simulink model "TestCase5_FromAero_RealWindTester"  (R2023a)
settings: Solver=ode4  StartTime=0.0  StopTime=120  FixedStep=0.01  RelTol=1e-3
values from neighbouring files (symbols this model uses):
  a0_All = [a0_s2 a0_s3 a0_s4 a0_s5]    [aeroProperties.m]
  aircraftMass = sum(componentMassesAndGeom(:,1))    [aircraftMassModel.m]
  AR_All = [AR_s2 AR_s3 AR_s4 AR_s5]    [DefineAircraftGeometry.m]
  c_All = [c_s2 c_s3 c_s4 c_s5]    [DefineAircraftGeometry.m]
  CD0_All = [CD0_s2 CD0_s3 CD0_s4 CD0_s5]    [aeroProperties.m]
  CDa_All = [CDa_s2 CDa_s3 CDa_s4 CDa_s5]    [aeroProperties.m]
  CG = [x_B_B_cmR y_B_B_cmR z_B_B_cmR]    [aircraftMassModel.m]
  CL0_All = [CL0_s2 CL0_s3 CL0_s4 CL0_s5]    [aeroProperties.m]
  CL_alpha_All = [CL_alpha_s2 CL_alpha_s3 CL_alpha_s4 CL_alpha_s5]    [aeroProperties.m]
  CM0_All = [CM0_s2 CM0_s3 CM0_s4 CM0_s5]    [aeroProperties.m]
  CMa_All = [CMa_s2 CMa_s3 CMa_s4 CMa_s5]    [aeroProperties.m]
  e_All = [e_s2 e_s3 e_s4 e_s5]    [aeroProperties.m]
  iAll = [i_s2 i_s3 i_s4 i_s5]    [aeroProperties.m]
  n_s2 = [0; 0; -1]    [aeroProperties.m]
  n_s3 = [0; 1; 0]    [aeroProperties.m]
  n_s4 = [0; 0; -1]    [aeroProperties.m]
  n_s5 = [0; 0; -1]    [aeroProperties.m]
  nAll = [n_s2 n_s3 n_s4 n_s5]    [aeroProperties.m]
  S_All = [S_s2 S_s3 S_s4 S_s5]    [DefineAircraftGeometry.m]
  x_horStab_B_B = [horStab_xLoc+0.25*c_s2 horStab_yLoc horStab_zLoc]    [aircraftMassModel.m]
  x_leftWingandServo_B_B = [leftWingandServo_xLoc+0.25*c_s5 leftWingandServo_yLoc leftWingandServo_zLoc]    [aircraftMassModel.m]
  x_rightWingandServo_B_B = [rightWingandServo_xLoc+0.25*c_s4 rightWingandServo_yLoc rightWingandServo_zLoc]    [aircraftMassModel.m]
  x_vertStab_B_B = [vertStab_xLoc+0.25*c_s3 vertStab_yLoc vertStab_zLoc]    [aircraftMassModel.m]
undefined symbols (not defined in the file or in its folder): earthRadius
libraries: matrix_library x6, simulink_extras x4, aerolibfltsims x2, aerolibtransform2 x1, aerolibutil x1, neural x1, sharedtransform x1
settings Model: Creator=fahee  LastModifiedBy=fahee

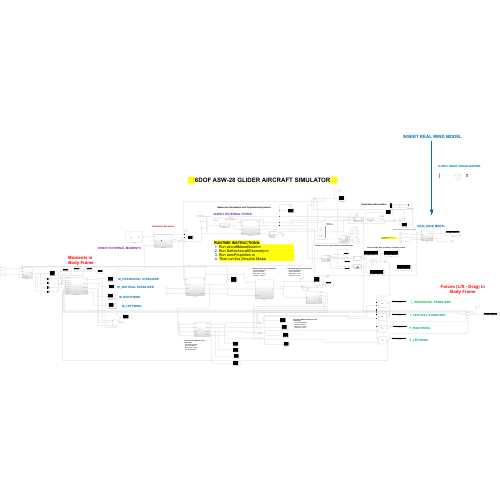
[thumbnail: Simulink's stored preview of the top-level diagram]
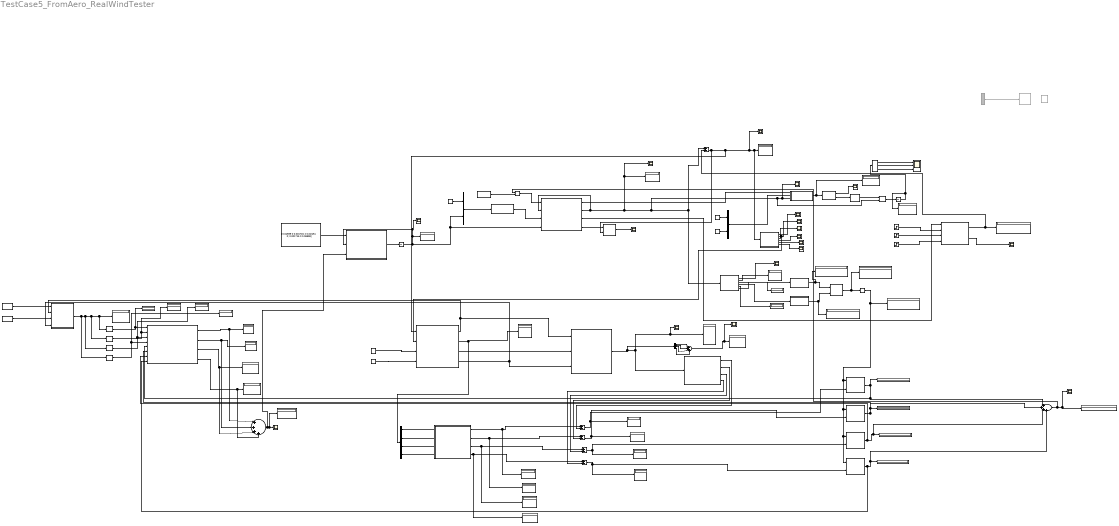
== system TestCase5_FromAero_RealWindTester ==
  note: FLIGHT GEAR VISUALIZATION
  note: v_N = C_N/B*v_B
  note: pure AKA null quaternion
      | vector part comes from rotational dynamics (omega)
  note: intersection of equator and prime meridian
  note: INSERT EXTERNAL FORCE
  note: 6DOF ASW-28 GLIDER AIRCRAFT SIMULATOR
  note: F_HORIZONTAL STABILIZER
  note: w_B/I
  note: w_B/I_dot
  note: Rotational Dynamics
  note: Translational Kinematics
  note: Latitude and Longitude (NED)
  note: Quaternion Kinematics and Translational Dynamics
  note: Calculate Airspeed, Angle of Attack and SideSlip Angle
  note: Calculate FORCE in Wind for each component
      | - Horzontal Stabilizer
      | - Vertical Stabilizer
      | - Right Wing + Servo
      | - Left Wing + Servo
  note: Calculate Drag for each component:
      | - Horzontal Stabilizer
      | - Vertical Stabilizer
      | - Right Wing + Servo
      | - Left Wing + Servo
  note: Calculate DCMs, Body to Stability and Stability to Wind
  note: Forces (Lift - Drag) in Body Frame
  note: F_VERTICAL STABILIZER
  note: F_RIGHTWING
  note: F_LEFTWING
  note: M_HORIZONTAL STABILIZER
  note: Moments in
      | Body Frame
  note: M_LEFTWING
  note: M_RIGHTWING
  note: M_VERTICAL STABILIZER
  note: Calculate Lift in Wind for each component
      | - Horzontal Stabilizer
      | - Vertical Stabilizer
      | - Right Wing + Servo
      | - Left Wing + Servo
  note: INSERT EXTERNAL MOMENTS
  note: w_B/I
  note: Specific Force = F_B/aircraftMass
  note: Calculate Lift for each component:
      | - Horzontal Stabilizer
      | - Vertical Stabilizer
      | - Right Wing + Servo
      | - Left Wing + Servo
  note: Add wind in NED as step input (set to 0 as default)
  note: INSERT REAL WIND MODEL
  note: Enter Wind Velocity, x, y z components
  note: RUNTIME INSTRUCTIONS:
      | Run aircraftMassModel.m
      | Run DefineAircraftGeometry.m
      | Run aeroProperties.m
      | Then run this Simulink Model
  note: REAL WIND MODEL
  AircraftMass_kg : Constant  Value=aircraftMass/1000
  Body2Stability : MATLAB Function  TreatAsAtomicUnit=on
  C_B/W : Display
  C_W/B : Display
  Calc Vinf alpha and beta : Subsystem
  Calc Vinf alpha and beta - with wind : Subsystem
  Calcualte v_BA_NED : Subsystem
  Calculate DRAG : Subsystem
  Calculate LIFT : Subsystem
  Constant : Constant  Value=iAll
  Constant1 : Constant  Value=nAll
  Constant17 : Constant  Value=CM0_All
  Constant18 : Constant  Value=CMa_All
  DRAG : Display
  Demux : Demux  Outputs=3
  Demux1 : Demux
  Demux2 : Demux
  Direction Cosine Matrix ECEF to NED : aerolibtransform2/Direction Cosine Matrix ECEF to NED
  Display{,1..4,7,14} (7 alike) : Display
  Divide4 : Product  Inputs=*/
  ECEF to LLA : Subsystem
  F_HorStab_Body : Display
  F_LeftWing_Body : Display
  F_RightWing_Body : Display
  F_VertStab_Body : Display
  FlightGear Preconfigured 6DoF Animation : aerolibfltsims/FlightGear Preconfigured 6DoF Animation  Commented=on  xFlightGearVersion=v2019.1  DestinationIpAddress=127.0.0.1  DestinationPort=5502  SampleTime=1/30  packetVersion=24
  Force_HorStab_WindFrame : Display
  Force_LeftWing_Wind : Display
  Force_RightWing_Wind : Display
  Force_VertStab_WindFrame : Display
  Generate Run Script : aerolibfltsims/Generate Run Script  Commented=on  Architecture=Win64  dataFlow=Send  GeometryModelName=c172p  AirportId=KSFO  RunwayId=10L  InitialAltitude=7224  InitialHeading=113  OffsetDistance=4.72  OffsetAzimuth=0  InstallScenery=off  DisableShaders=on  OriginAddress=127.0.0.1  DestinationPort=5502  OriginPort=5505  LocalAddress=127.0.0.1  OutputFileName=runfg.bat  FlightGearBaseDirectory=C:\Program Files\FlightGear 2020.3
  Inertia Matrix : Constant  Value=[0.04939 0 0.001715; 0 0.02151 0; 0.001715 0 0.06998]
  Integrator : Integrator  InitialCondition=[0 0 0]
  Integrator3 : Integrator  InitialCondition=[earthRadius,0,0]
  LIFT : Display
  L_HorStab_Wind : Display
  L_LeftWing_Wind : Display
  L_RightWing_Wind : Display
  L_VertStab_Wind : Display
  Lift_Wind : Subsystem
  MATLAB Function1 : MATLAB Function  TreatAsAtomicUnit=on
  M_LeftWing_Wind : Display
  M_RightWing_Wind : Display
  M_horstab_wind : Display
  M_vertstab_wind : Display
  Matrix Multiply3 : Product  Multiplication=Matrix(*)
  Moment_HorStab_BodyFrame : Display
  Moment_LeftWing_BodyFrame : Display
  Moment_RightWing_BodyFrame : Display
  Moment_VertStab_BodyFrame : Display
  Moment_Wind : Subsystem
  Moment_WindFrame : Display
  Moments Wind to Body : Subsystem
  Mux2 : Mux  Commented=on  Inputs=2
  Mux3 : Mux  Inputs=2
  Mux6 : Mux  Inputs=2
  Product{1,10..13} (5 alike) : Product  Multiplication=Matrix(*)
  Real Wind : Subsystem
  Rotational Dynamics : Subsystem
  Rotational Kinematics : Subsystem
  Scope{,1,4..11,13..14} (12 alike) : Scope
  Scope_x_B/E_E_latlonmethod : Scope  NumInputPorts=3
  Selector : Selector  InputPortWidth=4  IndexOptions=Index vector (dialog)  Indices=[1]  OutputSizes=1
  Selector1 : Selector  InputPortWidth=4  IndexOptions=Index vector (dialog)  Indices=[2]  OutputSizes=1
  Selector2 : Selector  InputPortWidth=4  IndexOptions=Index vector (dialog)  Indices=[3]  OutputSizes=1
  Selector3 : Selector  InputPortWidth=4  IndexOptions=Index vector (dialog)  Indices=[4]  OutputSizes=1
  Split to Drag For Each Control Surface : Subsystem
  Subtract{,1..4} (5 alike) : Sum  Inputs=+-
  Sum : Sum  Inputs=|++++
  Sum2 : Sum  Inputs=|++++
  Sum3 : Sum  Inputs=|++++
  Translational Dynamics : Subsystem
  Transpose3 : Math  Operator=transpose
  V_Wind_X : Step  Time=0  After=0  SampleTime=0
  V_Wind_Y : Step  Time=0  After=0  SampleTime=0
  V_Wind_Z : Step  Time=0  After=0  SampleTime=0
  VectTransform - Body to ECEF : Subsystem
  Vinf : Display
  Vinf alpha beta : Scope
  Wind in Body Frame : Display
  angle of attack : Display
  lat-lon-altitude : Scope
  latitude : Constant  Value=0
  longitude : Constant  Value=0
  qw1 : Constant  Value=0
  sideslip : Display
  v_B/E_B - no Wind : Display
  v_BA_B : Scope
  v_BA_B - subtracting Wind : Display
  v_Body : Scope
  v_NED : Scope
  x_B/E_E : Display
  x_B/Edot : Scope
  wires:
  Direction Cosine Matrix ECEF to NED/1 -> Matrix Multiply3/1
  Translational Dynamics/1(eul_N/B_out) -> VectTransform - Body to ECEF/1(eulAngle_N/B)
  latitude/1 -> Mux6/1
  Mux6/1 -> VectTransform - Body to ECEF/2(lat-lon)
  Matrix Multiply3/1 -> Integrator3/1
  Integrator/1 -> Translational Dynamics/4(w_B/E), Mux3/2, Display/1, Scope/1, Rotational Dynamics/2(w_B/I)
  qw1/1 -> Mux3/1
  VectTransform - Body to ECEF/1(rECEF) -> ECEF to LLA/1(rECEF), x_B/E_E/1
  longitude/1 -> Mux6/2
  Integrator3/1 -> Demux/1, Display14/1
  Demux/1 -> Scope_x_B/E_E_latlonmethod/1  "x_B/E_E"
  Demux/2 -> Scope_x_B/E_E_latlonmethod/2  "y_B/E_E"
  Demux/3 -> Scope_x_B/E_E_latlonmethod/3  "z_B/E_E"
  Subtract1/1 -> Product10/2, Force_HorStab_WindFrame/1
  Subtract2/1 -> Product11/2, Force_VertStab_WindFrame/1
  Subtract3/1 -> Force_RightWing_Wind/1, Product12/2
  Subtract4/1 -> Product13/2, Force_LeftWing_Wind/1
  Transpose3/1 -> Product13/1, Product12/1, Product11/1, Product10/1, C_B/W/1
  Product10/1 -> Moments Wind to Body/5(F_HorStab_Body), Sum/1, F_HorStab_Body/1
  Product11/1 -> Moments Wind to Body/6(F_VertStab_Body), Sum/2, F_VertStab_Body/1
  Product12/1 -> Sum/3, F_RightWing_Body/1, Moments Wind to Body/7(F_RightWing_Body)
  Product13/1 -> Moments Wind to Body/8(F_LeftWing_Body), Sum/4, F_LeftWing_Body/1
  Selector/1 -> M_horstab_wind/1, Moments Wind to Body/1(M_horstab_wind)
  Selector1/1 -> M_vertstab_wind/1, Moments Wind to Body/2(M_vertstab_wind)
  Selector2/1 -> M_RightWing_Wind/1, Moments Wind to Body/3(M_RightWing_Wind)
  Selector3/1 -> Moments Wind to Body/4(M_LeftWing_Wind), M_LeftWing_Wind/1
  Inertia Matrix/1 -> Rotational Dynamics/1(J)
  Rotational Dynamics/1(w_B/I_dot) -> Integrator/1
  Sum/1 -> Divide4/1, Scope7/1, Display7/1
  Mux3/1 -> Rotational Kinematics/1(qNull)
  ECEF to LLA/1(LLA) -> lat-lon-altitude/1
  ECEF to LLA/2(LatLon) -> Direction Cosine Matrix ECEF to NED/1
  Calculate LIFT/1(alpha) -> Moment_Wind/2(alpha), Calculate DRAG/1(alpha)
  Calculate LIFT/4(LDM_CommonTerm) -> Moment_Wind/4(LDM_CommonTerm), Calculate DRAG/3(LDM_CommonTerm)
  Calculate LIFT/2(Lift) -> LIFT/1, Demux2/1
  Constant1/1 -> Calculate LIFT/3(normalVector)
  Constant/1 -> Calculate LIFT/4(incidenceAngle)
  Calculate DRAG/1(Drag) -> Demux1/1, Split to Drag For Each Control Surface/1(Drag_All), Scope13/1, DRAG/1
  Calculate LIFT/3(CL) -> Calculate DRAG/2(CL)
  Split to Drag For Each Control Surface/1(D_HorStab) -> Subtract1/2
  Split to Drag For Each Control Surface/2(D_VertStab) -> Subtract2/2
  Split to Drag For Each Control Surface/3(D_RightWing) -> Subtract3/2
  Split to Drag For Each Control Surface/4(D_LeftWing) -> Subtract4/2
  Demux2/1 -> Lift_Wind/1(L_HorStab)
  Demux2/2 -> Lift_Wind/2(L_VertStab)
  Demux2/3 -> Lift_Wind/3(L_RightWing)
  Demux2/4 -> Lift_Wind/4(L_LeftWing)
  Lift_Wind/1(L_HorStab_Wind) -> L_HorStab_Wind/1, Subtract1/1
  Lift_Wind/2(L_VertStab_Wind) -> L_VertStab_Wind/1, Subtract2/1
  Lift_Wind/3(L_RightWing_Wind) -> Subtract3/1, L_RightWing_Wind/1
  Lift_Wind/4(L_LeftWing_Wind) -> L_LeftWing_Wind/1, Subtract4/1
  Moment_Wind/1(M_Wind) -> Moment_WindFrame/1, Selector/1, Selector1/1, Selector2/1, Selector3/1
  Constant17/1 -> Moment_Wind/1(CM0)
  Constant18/1 -> Moment_Wind/3(CMa)
  Moments Wind to Body/2(M_vertstab_body) -> Sum3/2, Moment_VertStab_BodyFrame/1
  Moments Wind to Body/3(M_RightWing_body) -> Sum3/3, Moment_RightWing_BodyFrame/1
  Moments Wind to Body/4(M_LeftWing_body) -> Sum3/4, Moment_LeftWing_BodyFrame/1
  Moments Wind to Body/1(M_horstab_body) -> Sum3/1, Moment_HorStab_BodyFrame/1
  Sum3/1 -> Rotational Dynamics/3(M_ext), Display4/1, Scope1/1
  Body2Stability/1(C_SB) -> Display2/1, Product1/2
  Product1/1 -> Transpose3/1, C_W/B/1
  Calc Vinf alpha and beta/2(Vinf) -> Vinf/1
  Calc Vinf alpha and beta/3(beta_deg) -> sideslip/1
  Calc Vinf alpha and beta/1(Vinf_alpha_beta) -> Vinf alpha beta/1
  Calc Vinf alpha and beta/4(alpha_rad) -> Body2Stability/1(alpha)
  Calc Vinf alpha and beta/5(alpha_deg) -> angle of attack/1
  Calc Vinf alpha and beta/6(beta_rad) -> MATLAB Function1/1(beta)
  Mux2/1 -> FlightGear Preconfigured 6DoF Animation/1
  Demux1/1 -> Sum2/1
  Demux1/2 -> Sum2/2
  Demux1/3 -> Sum2/3
  Demux1/4 -> Sum2/4
  Sum2/1 -> Scope14/1, Display1/1
  MATLAB Function1/1(C_WS) -> Display3/1, Product1/1
  AircraftMass_kg/1 -> Divide4/2
  Divide4/1 -> Translational Dynamics/1(F_ext)
  Subtract/1 -> Calcualte v_BA_NED/2(v_BA_B), Calculate LIFT/1(v_BA_B), v_BA_B/1, Calc Vinf alpha and beta - with wind/1(v_B/E), v_BA_B - subtracting Wind/1
  Calc Vinf alpha and beta - with wind/1(Vinf_alpha_beta) -> Scope4/1
  Calc Vinf alpha and beta - with wind/2(Vinf) -> Calculate LIFT/2(mag_v_BA_B), Scope5/1
  Calc Vinf alpha and beta - with wind/3(beta_deg) -> Scope6/1
  Calc Vinf alpha and beta - with wind/4(alpha_rad) -> Scope8/1
  Calc Vinf alpha and beta - with wind/5(alpha_deg) -> Scope9/1
  Calc Vinf alpha and beta - with wind/6(beta_rad) -> Scope10/1
  Real Wind/1(V_Wind_Body_Display) -> Subtract/2, Wind in Body Frame/1
  V_Wind_X/1 -> Real Wind/2(V_Wind_X)
  V_Wind_Y/1 -> Real Wind/3(V_Wind_Y)
  V_Wind_Z/1 -> Real Wind/4(V_Wind_Z)
  Real Wind/2(V_Wind_Body_Plot) -> Scope11/1
  Translational Dynamics/2(v_B/E) -> Translational Dynamics/2(v_B/E_In), v_B/E_B - no Wind/1, v_Body/1, Matrix Multiply3/2, x_B/Edot/1, VectTransform - Body to ECEF/3(x_B/Edot_B), Calc Vinf alpha and beta/1(v_B/E), Subtract/1
  Rotational Kinematics/1(q_B/N) -> Translational Dynamics/3(q_B/N)
  Translational Dynamics/3(C_B/N) -> Real Wind/1(C_B/N)
  Calcualte v_BA_NED/1(v_BA_N) -> v_NED/1
  Translational Dynamics/4(C_N/B) -> Calcualte v_BA_NED/1(C_N/B)

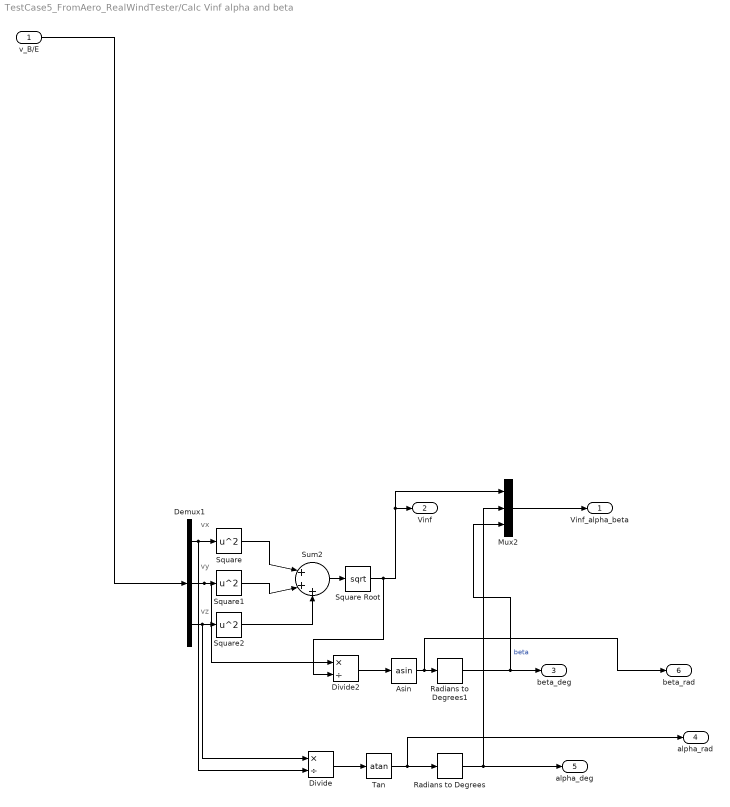
== system TestCase5_FromAero_RealWindTester/Calc Vinf alpha and beta ==
  note: vx
  note: vy
  note: vz
  v_B/E : Inport
  Asin : Trigonometry  Operator=asin
  Demux1 : Demux  Outputs=3
  Divide : Product  Inputs=*/
  Divide2 : Product  Inputs=*/
  Mux2 : Mux  Inputs=3
  Radians to Degrees : simulink_extras/Transformations/Radians to Degrees
  Radians to Degrees1 : simulink_extras/Transformations/Radians to Degrees
  Square : Math  Operator=square
  Square Root : Sqrt
  Square1 : Math  Operator=square
  Square2 : Math  Operator=square
  Sum2 : Sum  Inputs=|+++
  Tan : Trigonometry  Operator=atan
  Vinf_alpha_beta : Outport
  Vinf : Outport  Port=2
  beta_deg : Outport  Port=3
  alpha_rad : Outport  Port=4
  alpha_deg : Outport  Port=5
  beta_rad : Outport  Port=6
  wires:
  Demux1/3 -> Divide/1, Square2/1
  Square/1 -> Sum2/1
  Tan/1 -> alpha_rad/1, Radians to Degrees/1
  Mux2/1 -> Vinf_alpha_beta/1
  Demux1/2 -> Divide2/1, Square1/1
  Radians to Degrees1/1 -> beta_deg/1, Mux2/3  "beta"
  Square1/1 -> Sum2/2
  Divide2/1 -> Asin/1
  Sum2/1 -> Square Root/1
  Asin/1 -> beta_rad/1, Radians to Degrees1/1
  Divide/1 -> Tan/1
  Demux1/1 -> Square/1, Divide/2
  Radians to Degrees/1 -> alpha_deg/1, Mux2/2
  Square2/1 -> Sum2/3
  Square Root/1 -> Divide2/2, Mux2/1, Vinf/1
  v_B/E/1 -> Demux1/1

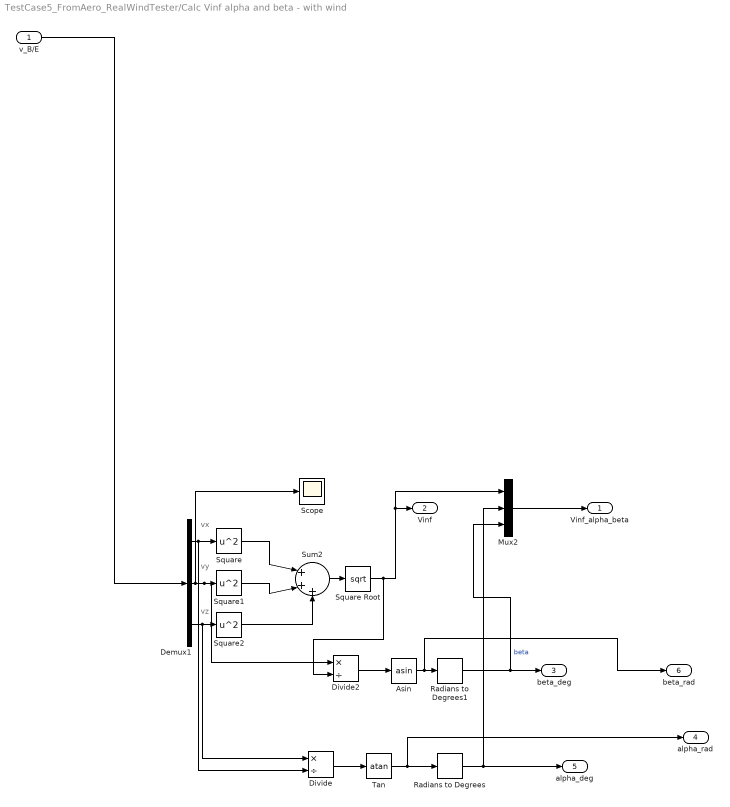
== system TestCase5_FromAero_RealWindTester/Calc Vinf alpha and beta - with wind ==
  note: vx
  note: vy
  note: vz
  v_B/E : Inport
  Asin : Trigonometry  Operator=asin
  Demux1 : Demux  Outputs=3
  Divide : Product  Inputs=*/
  Divide2 : Product  Inputs=*/
  Mux2 : Mux  Inputs=3
  Radians to Degrees : simulink_extras/Transformations/Radians to Degrees
  Radians to Degrees1 : simulink_extras/Transformations/Radians to Degrees
  Scope : Scope
  Square : Math  Operator=square
  Square Root : Sqrt
  Square1 : Math  Operator=square
  Square2 : Math  Operator=square
  Sum2 : Sum  Inputs=|+++
  Tan : Trigonometry  Operator=atan
  Vinf_alpha_beta : Outport
  Vinf : Outport  Port=2
  beta_deg : Outport  Port=3
  alpha_rad : Outport  Port=4
  alpha_deg : Outport  Port=5
  beta_rad : Outport  Port=6
  wires:
  Demux1/3 -> Divide/1, Square2/1
  Square/1 -> Sum2/1
  Tan/1 -> alpha_rad/1, Radians to Degrees/1
  Mux2/1 -> Vinf_alpha_beta/1
  Demux1/2 -> Divide2/1, Square1/1, Scope/1
  Radians to Degrees1/1 -> beta_deg/1, Mux2/3  "beta"
  Square1/1 -> Sum2/2
  Divide2/1 -> Asin/1
  Sum2/1 -> Square Root/1
  Asin/1 -> beta_rad/1, Radians to Degrees1/1
  Divide/1 -> Tan/1
  Demux1/1 -> Square/1, Divide/2
  Radians to Degrees/1 -> alpha_deg/1, Mux2/2
  Square2/1 -> Sum2/3
  Square Root/1 -> Divide2/2, Mux2/1, Vinf/1
  v_B/E/1 -> Demux1/1

== system TestCase5_FromAero_RealWindTester/Calcualte v_BA_NED ==
  C_N/B : Inport
  v_BA_B : Inport  Port=2
  Product24 : Product  Multiplication=Matrix(*)
  v_BA_N : Outport
  wires:
  Product24/1 -> v_BA_N/1
  v_BA_B/1 -> Product24/2
  C_N/B/1 -> Product24/1

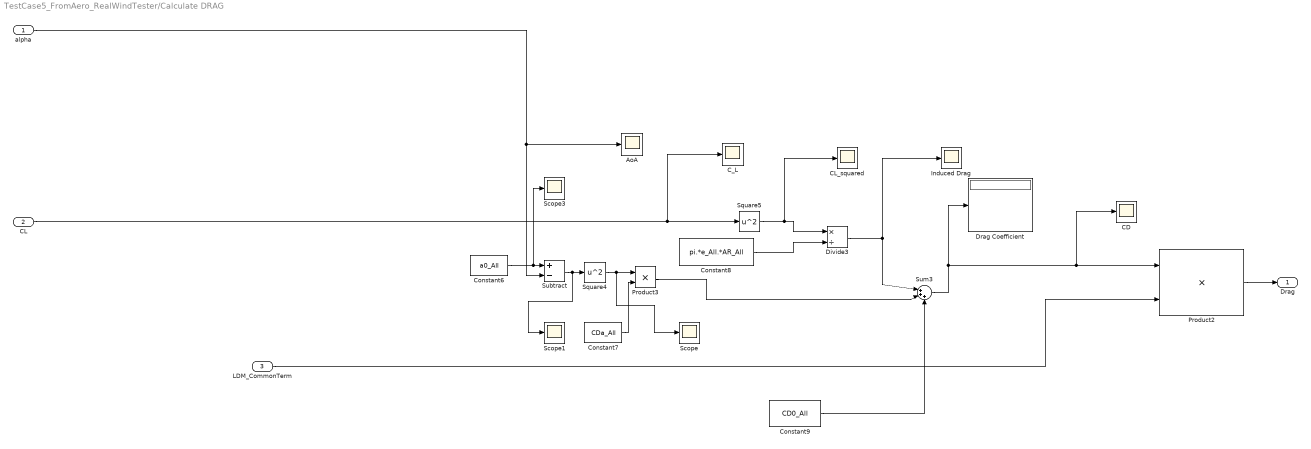
== system TestCase5_FromAero_RealWindTester/Calculate DRAG ==
  alpha : Inport
  CL : Inport  Port=2
  LDM_CommonTerm : Inport  Port=3
  AoA : Scope
  CD : Scope
  CL_squared : Scope
  C_L : Scope
  Constant6 : Constant  Value=a0_All
  Constant7 : Constant  Value=CDa_All
  Constant8 : Constant  Value=pi.*e_All.*AR_All
  Constant9 : Constant  Value=CD0_All
  Divide3 : Product  Inputs=*/
  Drag Coefficient : Display
  Induced Drag : Scope
  Product2 : Product
  Product3 : Product
  Scope : Scope
  Scope1 : Scope
  Scope3 : Scope
  Square4 : Math  Operator=square
  Square5 : Math  Operator=square
  Subtract : Sum  Inputs=+-
  Sum3 : Sum  Inputs=|+++
  Drag : Outport
  wires:
  Subtract/1 -> Scope1/1, Square4/1
  LDM_CommonTerm/1 -> Product2/2
  Constant6/1 -> Scope3/1, Subtract/1
  Constant7/1 -> Product3/2
  Product3/1 -> Sum3/2
  Square4/1 -> Scope/1, Product3/1
  Divide3/1 -> Sum3/1, Induced Drag/1
  Sum3/1 -> Drag Coefficient/1, CD/1, Product2/1
  Constant9/1 -> Sum3/3
  Square5/1 -> CL_squared/1, Divide3/1
  Constant8/1 -> Divide3/2
  Product2/1 -> Drag/1
  alpha/1 -> Subtract/2, AoA/1
  CL/1 -> C_L/1, Square5/1

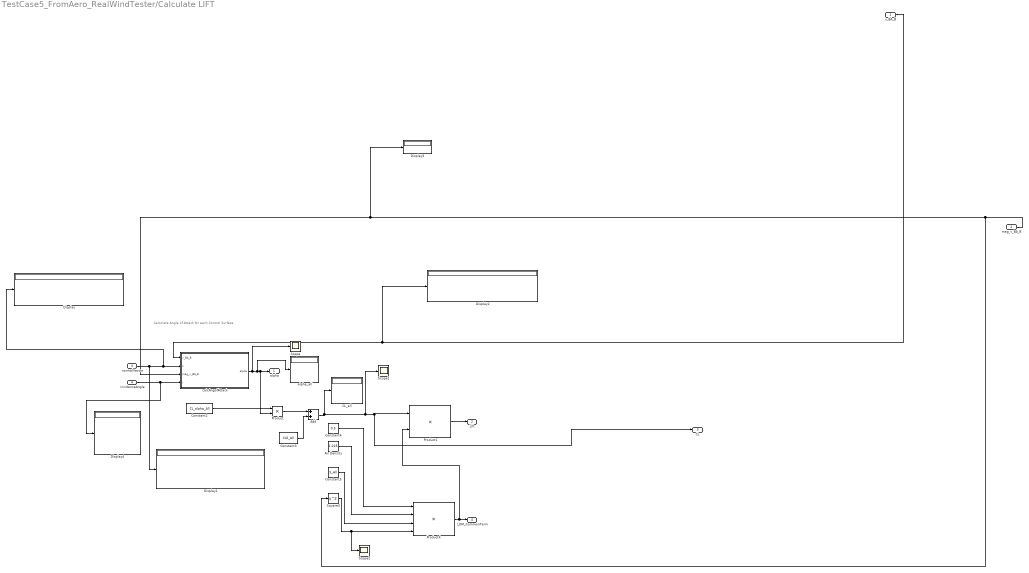
== system TestCase5_FromAero_RealWindTester/Calculate LIFT ==
  note: Calculate Angle of Attack for each Control Surface
  v_BA_B : Inport
  mag_v_BA_B : Inport  Port=2
  normalVector : Inport  Port=3
  incidenceAngle : Inport  Port=4
  Add : Sum
  Air Density : Constant  Value=1.225
  CL_all : Display
  Constant2 : Constant  Value=CL_alpha_All
  Constant3 : Constant  Value=CL0_All
  Constant4 : Constant  Value=0.5
  Constant5 : Constant  Value=S_All
  Display{,1..4} (5 alike) : Display
  Product : Product
  Product1 : Product
  Product4 : Product  Inputs=4
  Scope : Scope
  Scope1 : Scope
  Scope2 : Scope
  Square3 : Math  Operator=square
  alpha_all : Display
  calcAngofAttack : MATLAB Function  TreatAsAtomicUnit=on
  alpha : Outport
  Lift : Outport  Port=2
  CL : Outport  Port=3
  LDM_CommonTerm : Outport  Port=4
  wires:
  Air Density/1 -> Product4/2
  Constant3/1 -> Add/2
  incidenceAngle/1 -> Display4/1, calcAngofAttack/4(i)
  Constant5/1 -> Product4/3
  Constant4/1 -> Product4/1
  Add/1 -> Scope1/1, Product1/1, CL/1, CL_all/1
  normalVector/1 -> Display1/1, Display/1, calcAngofAttack/2(n)
  Square3/1 -> Scope2/1, Product4/4
  Product/1 -> Add/1
  Constant2/1 -> Product/1
  mag_v_BA_B/1 -> Square3/1, Display3/1, calcAngofAttack/3(mag_v_BA_B)
  calcAngofAttack/1(alpha) -> Scope/1, alpha_all/1, alpha/1, Product/2
  Product4/1 -> Product1/2, LDM_CommonTerm/1
  Product1/1 -> Lift/1
  v_BA_B/1 -> Display2/1, calcAngofAttack/1(v_BA_B)

== system TestCase5_FromAero_RealWindTester/ECEF to LLA ==
  note: x_B/Edot_B
  rECEF : Inport
  ECEF Position to LLA : ECEF2LLA  ptype=Custom  R=earthRadius
  Mux4 : Mux  Inputs=2
  altitude : Display
  lat & lon : Display
  LLA : Outport
  LatLon : Outport  Port=2
  wires:
  Mux4/1 -> LLA/1
  ECEF Position to LLA/2 -> Mux4/2, altitude/1
  ECEF Position to LLA/1 -> LatLon/1, Mux4/1, lat & lon/1
  rECEF/1 -> ECEF Position to LLA/1

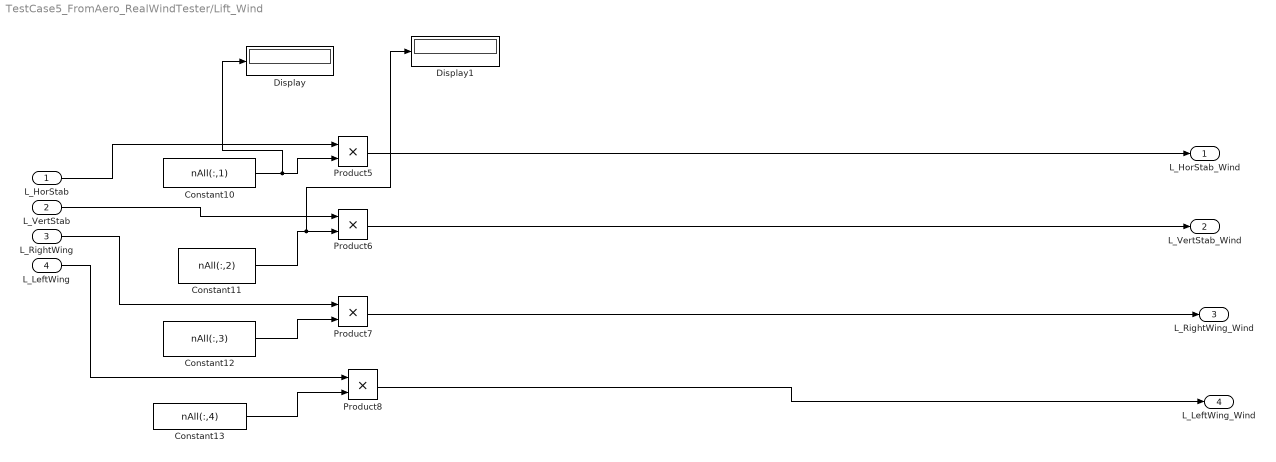
== system TestCase5_FromAero_RealWindTester/Lift_Wind ==
  L_HorStab : Inport
  L_VertStab : Inport  Port=2
  L_RightWing : Inport  Port=3
  L_LeftWing : Inport  Port=4
  Constant10 : Constant  Value=nAll(:,1)
  Constant11 : Constant  Value=nAll(:,2)
  Constant12 : Constant  Value=nAll(:,3)
  Constant13 : Constant  Value=nAll(:,4)
  Display : Display
  Display1 : Display
  Product{5..8} (4 alike) : Product
  L_HorStab_Wind : Outport
  L_VertStab_Wind : Outport  Port=2
  L_RightWing_Wind : Outport  Port=3
  L_LeftWing_Wind : Outport  Port=4
  wires:
  L_LeftWing/1 -> Product8/1
  L_VertStab/1 -> Product6/1
  Constant11/1 -> Display1/1, Product6/2
  Constant10/1 -> Display/1, Product5/2
  Constant13/1 -> Product8/2
  Constant12/1 -> Product7/2
  L_RightWing/1 -> Product7/1
  Product8/1 -> L_LeftWing_Wind/1
  L_HorStab/1 -> Product5/1
  Product7/1 -> L_RightWing_Wind/1
  Product6/1 -> L_VertStab_Wind/1
  Product5/1 -> L_HorStab_Wind/1

== system TestCase5_FromAero_RealWindTester/Moment_Wind ==
  CM0 : Inport
  alpha : Inport  Port=2
  CMa : Inport  Port=3
  LDM_CommonTerm : Inport  Port=4
  Constant19 : Constant  Value=c_All
  Moment Coefficient : Display
  Product14 : Product
  Product15 : Product  Inputs=3
  Sum4 : Sum  Inputs=|++
  M_Wind : Outport
  wires:
  Sum4/1 -> Product15/2, Moment Coefficient/1
  Constant19/1 -> Product15/3
  LDM_CommonTerm/1 -> Product15/1
  alpha/1 -> Product14/2
  CM0/1 -> Sum4/1
  CMa/1 -> Product14/1
  Product15/1 -> M_Wind/1
  Product14/1 -> Sum4/2

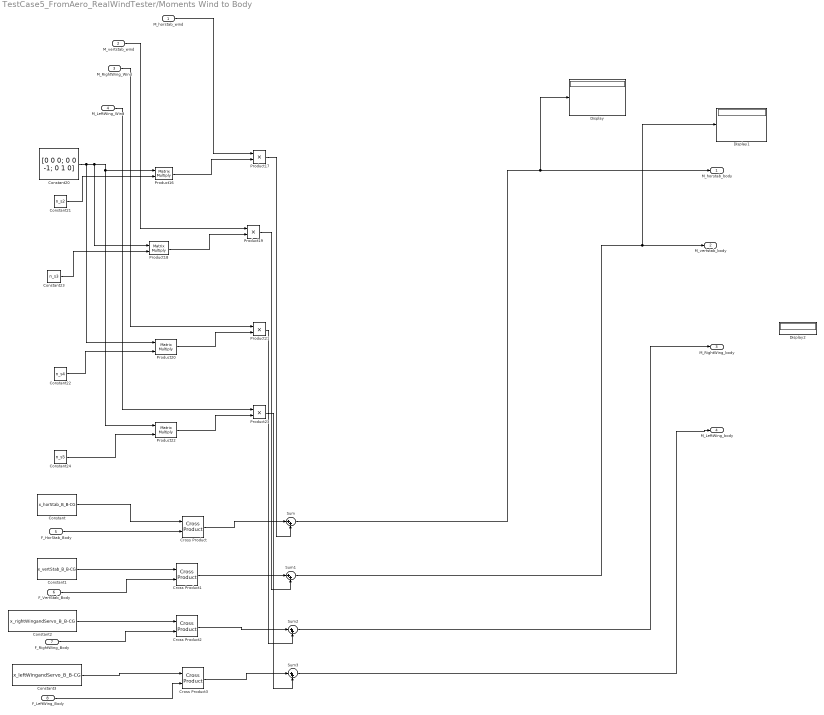
== system TestCase5_FromAero_RealWindTester/Moments Wind to Body ==
  M_horstab_wind : Inport
  M_vertstab_wind : Inport  Port=2
  M_RightWing_Wind : Inport  Port=3
  M_LeftWing_Wind : Inport  Port=4
  F_HorStab_Body : Inport  Port=5
  F_VertStab_Body : Inport  Port=6
  F_RightWing_Body : Inport  Port=7
  F_LeftWing_Body : Inport  Port=8
  Constant : Constant  Value=x_horStab_B_B-CG
  Constant1 : Constant  Value=x_vertStab_B_B-CG
  Constant2 : Constant  Value=x_rightWingandServo_B_B-CG
  Constant20 : Constant  Value=[0 0 0; 0 0 -1; 0 1 0]  VectorParams1D=off  SampleTime=-1
  Constant21 : Constant  Value=n_s2
  Constant22 : Constant  Value=n_s4
  Constant23 : Constant  Value=n_s3
  Constant24 : Constant  Value=n_s5
  Constant3 : Constant  Value=x_leftWingandServo_B_B-CG
  Cross Product{,1..3} (4 alike) : matrix_library/Cross Product
  Display : Display
  Display1 : Display
  Display2 : Display
  Product{16,18,20,22} (4 alike) : Product  Multiplication=Matrix(*)
  Product{17,19,21,23} (4 alike) : Product
  Sum{,1..3} (4 alike) : Sum  Inputs=|++
  M_horstab_body : Outport
  M_vertstab_body : Outport  Port=2
  M_RightWing_body : Outport  Port=3
  M_LeftWing_body : Outport  Port=4
  wires:
  Constant22/1 -> Product20/2
  Constant20/1 -> Product20/1, Product18/1, Product22/1, Product16/1
  Product18/1 -> Product19/2
  Constant21/1 -> Product16/2
  Constant24/1 -> Product22/2
  Constant23/1 -> Product18/2
  M_vertstab_wind/1 -> Product19/1
  Product22/1 -> Product23/2
  Product20/1 -> Product21/2
  M_horstab_wind/1 -> Product17/1
  Product16/1 -> Product17/2
  M_RightWing_Wind/1 -> Product21/1
  M_LeftWing_Wind/1 -> Product23/1
  Constant/1 -> Cross Product/1
  F_HorStab_Body/1 -> Cross Product/2
  Cross Product/1 -> Sum/1
  Product17/1 -> Sum/2
  Sum/1 -> Display/1, M_horstab_body/1
  Constant1/1 -> Cross Product1/1
  F_VertStab_Body/1 -> Cross Product1/2
  Cross Product1/1 -> Sum1/1
  Product19/1 -> Sum1/2
  Sum1/1 -> Display1/1, M_vertstab_body/1
  Constant2/1 -> Cross Product2/1
  F_RightWing_Body/1 -> Cross Product2/2
  Cross Product2/1 -> Sum2/1
  Product21/1 -> Sum2/2
  Sum2/1 -> M_RightWing_body/1
  Constant3/1 -> Cross Product3/1
  F_LeftWing_Body/1 -> Cross Product3/2
  Cross Product3/1 -> Sum3/1
  Product23/1 -> Sum3/2
  Sum3/1 -> M_LeftWing_body/1

== system TestCase5_FromAero_RealWindTester/Real Wind ==
  C_B/N : Inport
  V_Wind_X : Inport  Port=2
  V_Wind_Y : Inport  Port=3
  V_Wind_Z : Inport  Port=4
  Mux4 : Mux  Inputs=3
  Product : Product  Multiplication=Matrix(*)
  V_Wind_Body_Display : Outport
  V_Wind_Body_Plot : Outport  Port=2
  wires:
  Mux4/1 -> V_Wind_Body_Plot/1, Product/2
  Product/1 -> V_Wind_Body_Display/1
  C_B/N/1 -> Product/1
  V_Wind_Y/1 -> Mux4/2
  V_Wind_X/1 -> Mux4/1
  V_Wind_Z/1 -> Mux4/3

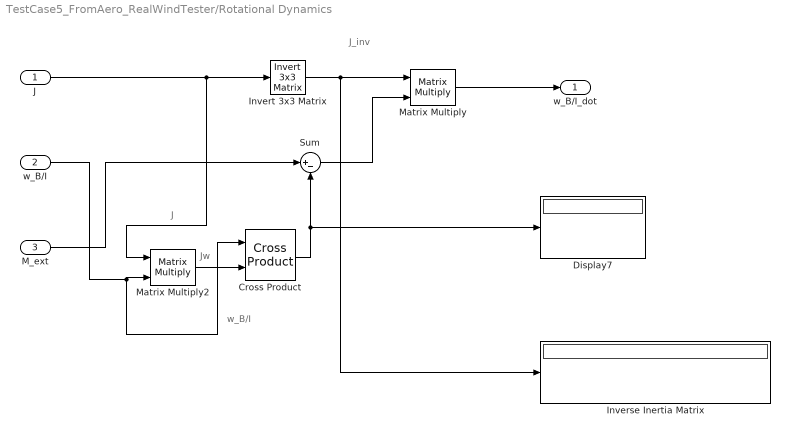
== system TestCase5_FromAero_RealWindTester/Rotational Dynamics ==
  note: J
  note: Jw
  note: J_inv
  note: w_B/I
  J : Inport
  w_B/I : Inport  Port=2
  M_ext : Inport  Port=3
  Cross Product : matrix_library/Cross Product
  Display7 : Display
  Inverse Inertia Matrix : Display
  Invert 3x3 Matrix : aerolibutil/Invert  3x3 Matrix
  Matrix Multiply : Product  Multiplication=Matrix(*)
  Matrix Multiply2 : Product  Multiplication=Matrix(*)
  Sum : Sum  Inputs=|+-
  w_B/I_dot : Outport
  wires:
  Sum/1 -> Matrix Multiply/2
  Cross Product/1 -> Sum/2, Display7/1
  w_B/I/1 -> Cross Product/1, Matrix Multiply2/2
  Matrix Multiply/1 -> w_B/I_dot/1
  J/1 -> Matrix Multiply2/1, Invert 3x3 Matrix/1
  M_ext/1 -> Sum/1
  Matrix Multiply2/1 -> Cross Product/2
  Invert 3x3 Matrix/1 -> Matrix Multiply/1, Inverse Inertia Matrix/1

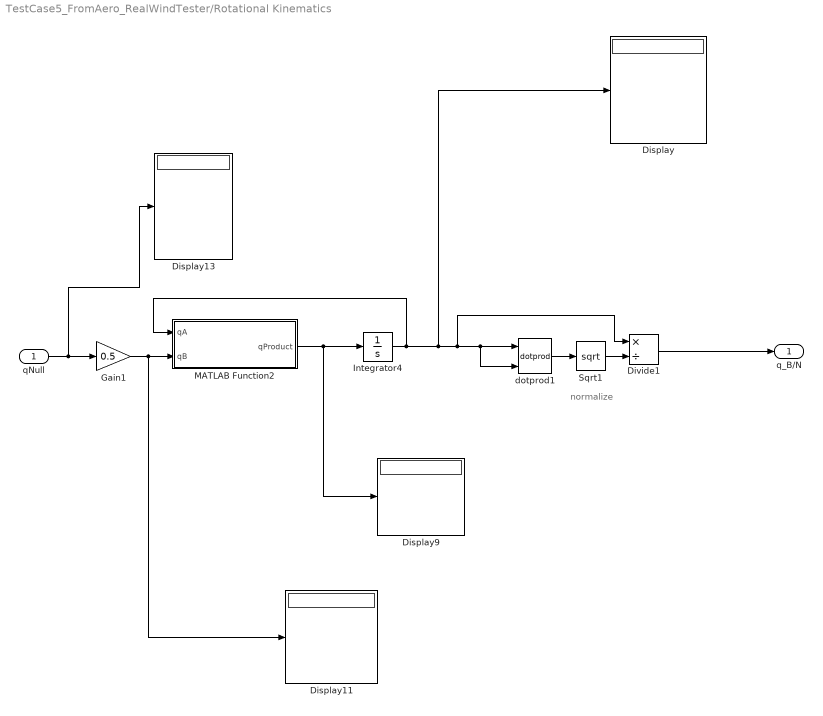
== system TestCase5_FromAero_RealWindTester/Rotational Kinematics ==
  note: normalize
  qNull : Inport
  Display{,9,11,13} (4 alike) : Display
  Divide1 : Product  Inputs=*/
  Gain1 : Gain  Gain=0.5
  Integrator4 : Integrator  InitialCondition=[0.9993 0 -0.03804 0]'
  MATLAB Function2 : MATLAB Function  TreatAsAtomicUnit=on
  Sqrt1 : Sqrt
  dotprod1 : neural/Weight Functions/dotprod
  q_B/N : Outport
  wires:
  Integrator4/1 -> Display/1, Divide1/1, dotprod1/2, dotprod1/1, MATLAB Function2/1(qA)
  dotprod1/1 -> Sqrt1/1
  Gain1/1 -> MATLAB Function2/2(qB), Display11/1
  qNull/1 -> Gain1/1, Display13/1
  MATLAB Function2/1(qProduct) -> Integrator4/1, Display9/1
  Sqrt1/1 -> Divide1/2
  Divide1/1 -> q_B/N/1

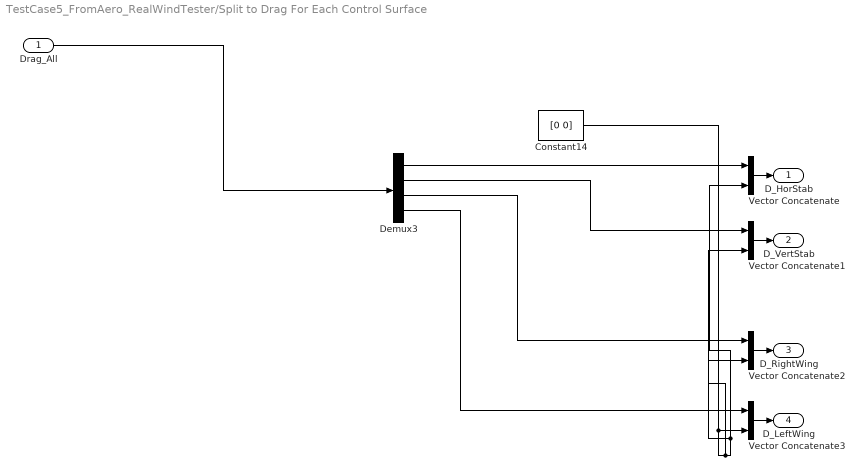
== system TestCase5_FromAero_RealWindTester/Split to Drag For Each Control Surface ==
  Drag_All : Inport
  Constant14 : Constant  Value=[0 0]
  Demux3 : Demux
  Vector Concatenate{,1..3} (4 alike) : Concatenate
  D_HorStab : Outport
  D_VertStab : Outport  Port=2
  D_RightWing : Outport  Port=3
  D_LeftWing : Outport  Port=4
  wires:
  Vector Concatenate1/1 -> D_VertStab/1
  Demux3/3 -> Vector Concatenate2/1
  Constant14/1 -> Vector Concatenate1/2, Vector Concatenate2/2, Vector Concatenate/2, Vector Concatenate3/2
  Vector Concatenate2/1 -> D_RightWing/1
  Demux3/2 -> Vector Concatenate1/1
  Drag_All/1 -> Demux3/1
  Demux3/1 -> Vector Concatenate/1
  Demux3/4 -> Vector Concatenate3/1
  Vector Concatenate/1 -> D_HorStab/1
  Vector Concatenate3/1 -> D_LeftWing/1

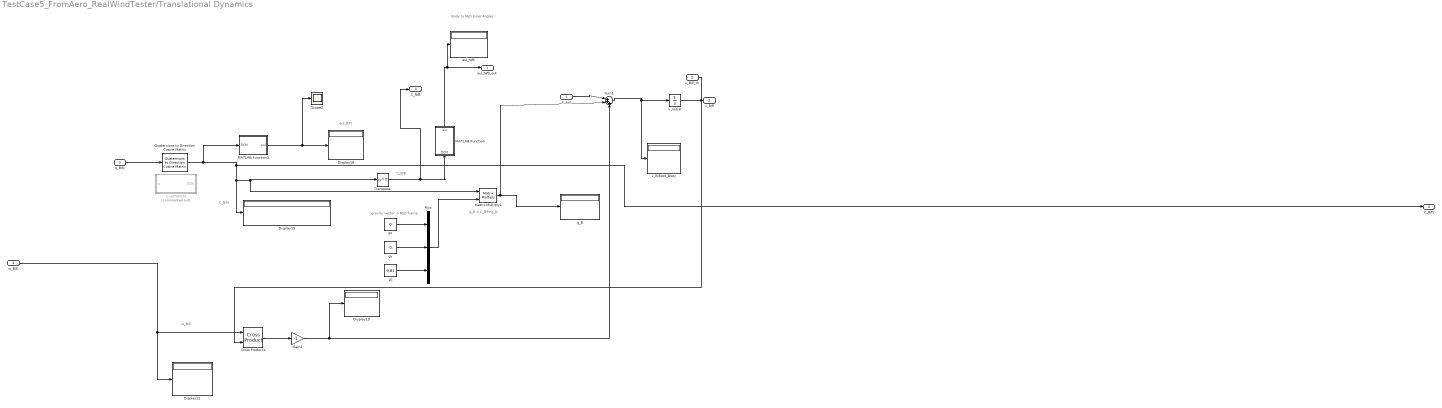
== system TestCase5_FromAero_RealWindTester/Translational Dynamics ==
  note: gravity vector in NED frame
  note: C_N/B
  note: eul_B/N
  note: C_B/N
  note: g_B = C_B/N*g_N
  note: Body to NED Euler Angles
  note: w_B/E
  F_ext : Inport
  v_B/E_In : Inport  Port=2
  q_B/N : Inport  Port=3
  w_B/E : Inport  Port=4
  Cross Product1 : matrix_library/Cross Product
  Display{12,15,18..19} (4 alike) : Display
  Gain2 : Gain  Gain=-1
  MATLAB Function : MATLAB Function  TreatAsAtomicUnit=on
  MATLAB Function3 : MATLAB Function  TreatAsAtomicUnit=on
  Matrix Multiply1 : Product  Multiplication=Matrix(*)
  Mux : Mux  Inputs=3
  QuatToDCM : MATLAB Function  Commented=on  TreatAsAtomicUnit=on
  Quaternions to Direction Cosine Matrix : sharedtransform/Quaternions to  Direction Cosine Matrix  aMode=aMode
      settings: LibrarySourceBlock=|
      | aerolibtransform2/Quaternions to
      | Direction Cosine Matrix
  Scope3 : Scope
  Sum1 : Sum  Inputs=|+++
  Transpose : Math  Operator=transpose
  eul_N/B : Display
  g_B : Display
  gx : Constant  Value=0
  gy : Constant  Value=0
  gz : Constant  Value=9.81
  v_B/Edot_Body : Display
  v_Initial : Integrator  InitialCondition=[13.17 0 -0.1809]
  eul_N/B_out : Outport
  v_B/E : Outport  Port=2
  C_B/N : Outport  Port=3
  C_N/B : Outport  Port=4
  wires:
  Quaternions to Direction Cosine Matrix/1 -> MATLAB Function3/1(DCM), Display15/1, Transpose/1, Matrix Multiply1/1, C_B/N/1
  gy/1 -> Mux/2
  w_B/E/1 -> Cross Product1/1, Display12/1
  Sum1/1 -> v_B/Edot_Body/1, v_Initial/1
  q_B/N/1 -> Quaternions to Direction Cosine Matrix/1
  Gain2/1 -> Sum1/3, Display19/1
  Cross Product1/1 -> Gain2/1
  Transpose/1 -> C_N/B/1, MATLAB Function/1(DCM)
  Mux/1 -> Matrix Multiply1/2
  F_ext/1 -> Sum1/1
  MATLAB Function3/1(eul) -> Display18/1, Scope3/1
  Matrix Multiply1/1 -> Sum1/2, g_B/1
  gx/1 -> Mux/1
  gz/1 -> Mux/3
  v_Initial/1 -> v_B/E/1
  v_B/E_In/1 -> Cross Product1/2
  MATLAB Function/1(eul) -> eul_N/B/1, eul_N/B_out/1

== system TestCase5_FromAero_RealWindTester/VectTransform - Body to ECEF ==
  note: NED to ECEF
  eulAngle_N/B : Inport
  lat-lon : Inport  Port=2
  x_B/Edot_B : Inport  Port=3
  Body to ECEF : Subsystem
  Display : Display
  Integrator1 : Integrator  InitialCondition=[6.371e6 0 1577]
  Scope : Scope
  rECEF : Outport
  wires:
  Integrator1/1 -> Display/1, rECEF/1, Scope/1
  eulAngle_N/B/1 -> Body to ECEF/1(eulAngle_N/B)
  Body to ECEF/1(x_B/Edot_E) -> Integrator1/1
  lat-lon/1 -> Body to ECEF/2(lat-lon)
  x_B/Edot_B/1 -> Body to ECEF/3(x_B/Edot_B)

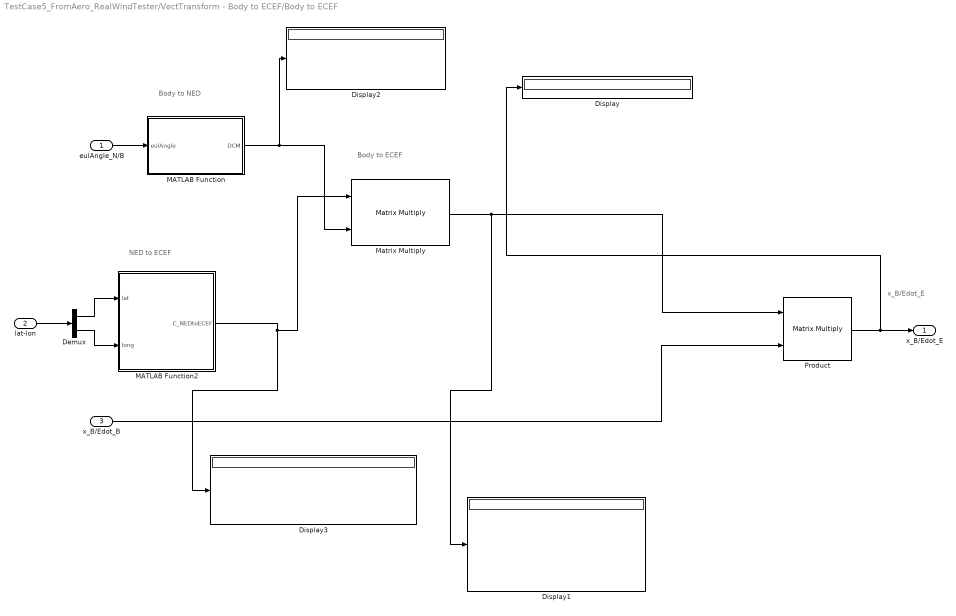
== system TestCase5_FromAero_RealWindTester/VectTransform - Body to ECEF/Body to ECEF ==
  note: NED to ECEF
  note: Body to NED
  note: x_B/Edot_E
  note: Body to ECEF
  eulAngle_N/B : Inport
  lat-lon : Inport  Port=2
  x_B/Edot_B : Inport  Port=3
  Demux : Demux  Outputs=2
  Display{,1..3} (4 alike) : Display
  MATLAB Function : MATLAB Function  TreatAsAtomicUnit=on
  MATLAB Function2 : MATLAB Function  TreatAsAtomicUnit=on
  Matrix Multiply : Product  Multiplication=Matrix(*)
  Product : Product  Multiplication=Matrix(*)
  x_B/Edot_E : Outport
  wires:
  Matrix Multiply/1 -> Display1/1, Product/1
  eulAngle_N/B/1 -> MATLAB Function/1(eulAngle)
  lat-lon/1 -> Demux/1
  x_B/Edot_B/1 -> Product/2
  Product/1 -> Display/1, x_B/Edot_E/1
  MATLAB Function2/1(C_NEDtoECEF) -> Display3/1, Matrix Multiply/1
  MATLAB Function/1(DCM) -> Display2/1, Matrix Multiply/2
  Demux/1 -> MATLAB Function2/1(lat)
  Demux/2 -> MATLAB Function2/2(long)

== matlab function TestCase5_FromAero_RealWindTester/Rotational Kinematics/MATLAB Function2 ==
  data: qA input; qProduct output; qB input
function qProduct = qMult(qA,qB)

%% qMult

% Description: This function is used to perform quaternion multiplication:
%            *************************************************************  
%               qA * qB = qProduct = [ qA(1)*qB(1) - (qA(2:4) dot qB(2:4)); 
%                                     (qA(1)*qB(2:4) + qB(1)*qA(2:4) +
%                                     qA(2:4) cross qB(2:4) ]
%            *************************************************************
% % Aircraft Control and Simulation Third Edition Page 46 Eq 1.8.-4
%
% Inputs:
%  qA - first quaternion in the form [qw qx qy qz]
%  qB - second quaternion in the form [qw qx qy qz]
%
% Output:
%  qProduct - the product of multiplying qA * qB [qw qx qy qz]

% if (norm(qA) ~= 1)
%     error('First quaternion inputted must have length 1. Invalid Quaternion. Try again.')
% end
% 
% if (norm(qB) ~= 1)
%     error('Second quaternion inputted must have length 1. Invalid Quaternion. Try again.')
% end

% Extract scalar components of each of the input quaternions
qA_w = qA(1);
qB_w = qB(1);

% Extract vector components of each of the input quaternions
qA_vect = qA(2:4);
qB_vect = qB(2:4);

% Calculate scalar component of the product of the two quaternions
% Aircraft Control and Simulation Third Edition Page 46 Eq 1.8.-4
qProd_w = (qA_w*qB_w - dot(qA_vect,qB_vect));

% Calculate vector components of the product of the two quaternions
% Aircraft Control and Simulation Third Edition Page 46 Eq 1.8.-4
qProd_vect = qA_w*qB_vect + qB_w*qA_vect + cross(qA_vect,qB_vect);

% Put scalar and vector products together to form qProduct
qProduct = [qProd_w; qProd_vect];

end

== matlab function TestCase5_FromAero_RealWindTester/Translational Dynamics/QuatToDCM ==
  data: q input; DCM output
function DCM = QuatToDCM(q)

%% QuatToDCM

% This function is used to convert quaternion to DCM

% if (norm(q) ~= 1)
%     error('First quaternion inputted must have length 1. Invalid Quaternion. Try again.')
% end

qw = q(1);
qx = q(2);
qy = q(3);
qz = q(4);

DCM_11 = qw^2 + qx^2 - qy^2 - qz^2;
DCM_12 = 2*(qx*qy + qz*qw);
DCM_13 = 2*(qx*qz - qy*qw);

DCM_21 = 2*(qx*qy - qz*qw);
DCM_22 = qw^2 - qx^2 + qy^2 - qz^2;
DCM_23 = 2*(qy*qz + qx*qw);

DCM_31 = 2*(qx*qz + qy*qw);
DCM_32 = 2*(qy*qz - qx*qw);
DCM_33 = qw^2 - qx^2 - qy^2 + qz^2;

DCM = [DCM_11 DCM_12 DCM_13; DCM_21 DCM_22 DCM_23; DCM_31 DCM_32 DCM_33];


end

== matlab function TestCase5_FromAero_RealWindTester/VectTransform - Body to ECEF/Body to ECEF/MATLAB Function2 ==
  data: lat input; C_NEDtoECEF output; long input
function C_NEDtoECEF = NEDtoECEF(lat,long)

Cy = [cos(lat) 0 -sin(lat); 0 1 0; sin(lat) 0 cos(lat)];
Cx = [1 0 0; 0 cos(-long) sin(-long); 0 -sin(long) cos(-long)];
Cy90 = [cos(pi/2) 0 -sin(pi/2); 0 1 0; sin(pi/2) 0 cos(pi/2)];

C_NEDtoECEF = Cy90*Cy*Cx;


end

== matlab function TestCase5_FromAero_RealWindTester/VectTransform - Body to ECEF/Body to ECEF/MATLAB Function ==
  data: eulAngle input; DCM output
function DCM = EulToDCM(eulAngle)

%% EulToDCM

% AME 532a HW 1 Problem 5a
% Faheem Chunara
% USC ID: 8660882618
% January 22, 2024
%
%  Description: This function converts Euler Angles (Roll-Pitch-Yaw) to Direction Cosine Matrix (DCM).
%
%  Input
%   eulAngle - Euler angles (Roll-Pitch-Yaw) (3x1) (radians)
%
%  Output
%   DCM - Direction Cosine Matrix (DCM) (3x3) 

% Extract Roll, Pitch, Yaw Euler angles and store to a variable
eul_1 = eulAngle(1); % Roll
eul_2 = eulAngle(2); % Pitch
eul_3 = eulAngle(3); % Yaw

% DCM x-axis rotation: R_x(angle) 
DCM_1 = [1 0 0; 0 cos(eul_1) sin(eul_1); 0 -sin(eul_1) cos(eul_1)]; 

% DCM y-axis rotation: R_y(angle) 
DCM_2 = [cos(eul_2) 0 -sin(eul_2); 0 1 0; sin(eul_2) 0 cos(eul_2)];

% DCM z-axis rotation: R_z(angle) 
DCM_3 = [cos(eul_3) sin(eul_3) 0; -sin(eul_3) cos(eul_3) 0; 0 0 1];

% DCM for rotation order XYZ (Rz*Rx*Ry) 
DCM = DCM_3*DCM_2*DCM_1;

end

== matlab function TestCase5_FromAero_RealWindTester/Calculate LIFT/calcAngofAttack ==
  data: v_BA_B input; alpha output; n input; mag_v_BA_B input; i input
function alpha = calcAngofAttack(v_BA_B,n,mag_v_BA_B,i)

% Description: Calculates angle of attack for each lifting body

% Inputs:
%  1. v_BA_B     - velocity in the body frame
%  2. n          - unit vector of vertical
%  3. mag_v_BA_B - magnitude of velocity in body frame
%  4. i          - incidence angle

% Outputs:
%  1. alpha      - angle of attack

alpha = zeros(length(n),1);

for k = 1:length(n)
    alpha(k) = i(k) - asin( dot(v_BA_B', n(:,k)) / mag_v_BA_B);
end

== matlab function TestCase5_FromAero_RealWindTester/Translational Dynamics/MATLAB Function3 ==
  data: DCM input; eul output
function eul = DCMToEul(DCM)

%% DCMToEul

% AME 532a HW 1 Problem 5b
% Faheem Chunara
% USC ID: 8660882618
% January 22, 2024
%
%  Description: This function converts a Direction Cosine Matrix (DCM) to
%  Euler Angles (ZYX) AKA (3-2-1) Rotation Sequence.
%
% Input
%  DCM - Direction cosine matrix AKA rotation matrix that you want to
%        convert to Euler Angles (3x3)
%
% Output
%  eul - Euler angles ZYX (3-2-1) (3x1) (radians)


% Calculate roll, pitch, yaw euler angles (Aircraft Control and Simulation
% Third Edition Page 12 - Euler Angles from the DCM)
roll = atan2(DCM(2,3),DCM(3,3));
pitch = -1*asin(DCM(1,3));
yaw = atan2(DCM(1,2),DCM(1,1));

% Put euler angles in one output variable
eul = [roll,pitch,yaw]';

end

== matlab function TestCase5_FromAero_RealWindTester/Body2Stability ==
  data: alpha input; C_SB output
function C_SB = Body2Stability(alpha)

% alpha must be in radians

C_SB = [cos(alpha) 0 sin(alpha); 0 1 0; -sin(alpha) 0 cos(alpha)];

end

== matlab function TestCase5_FromAero_RealWindTester/MATLAB Function1 ==
  data: beta input; C_WS output
function C_WS = Stability2Wind(beta)

C_WS = [cos(beta) sin(beta) 0; -sin(beta) cos(beta) 0; 0 0 1];

end

== matlab function TestCase5_FromAero_RealWindTester/Translational Dynamics/MATLAB Function ==
  data: DCM input; eul output
function eul = DCMToEul(DCM)

%% DCMToEul

% AME 532a HW 1 Problem 5b
% Faheem Chunara
% USC ID: 8660882618
% January 22, 2024
%
%  Description: This function converts a Direction Cosine Matrix (DCM) to
%  Euler Angles (ZYX) AKA (3-2-1) Rotation Sequence.
%
% Input
%  DCM - Direction cosine matrix AKA rotation matrix that you want to
%        convert to Euler Angles (3x3)
%
% Output
%  eul - Euler angles ZYX (3-2-1) (3x1) (radians)


% Calculate roll, pitch, yaw euler angles (Aircraft Control and Simulation
% Third Edition Page 12 - Euler Angles from the DCM)
roll = atan2(DCM(2,3),DCM(3,3));
pitch = -1*asin(DCM(1,3));
yaw = atan2(DCM(1,2),DCM(1,1));

% Put euler angles in one output variable
eul = [roll,pitch,yaw];

end
